simulink model "Appl_HeatAdj_CtrlModel"  (R2018b)
settings: configuration reference "CodeConfig_10_ms" (kept outside this file)
undefined symbols (not defined in the file): CAL_LEVEL3_TIMEOUT, CAL_SW_20min_TIMEOUT, D_1stLevel_36, D_2ndLevel_39, D_3rdLevel_45, D_3rdLevel_48, D_DRVHEAT_PID_D, D_DRVHEAT_PID_I, D_DRVHEAT_PID_P, D_HEAT_HEAT_DEF, D_SwsLevel_Temp, FALSE, TRUE
libraries: DareLib x111, simulink x1
(part 2 of 6)

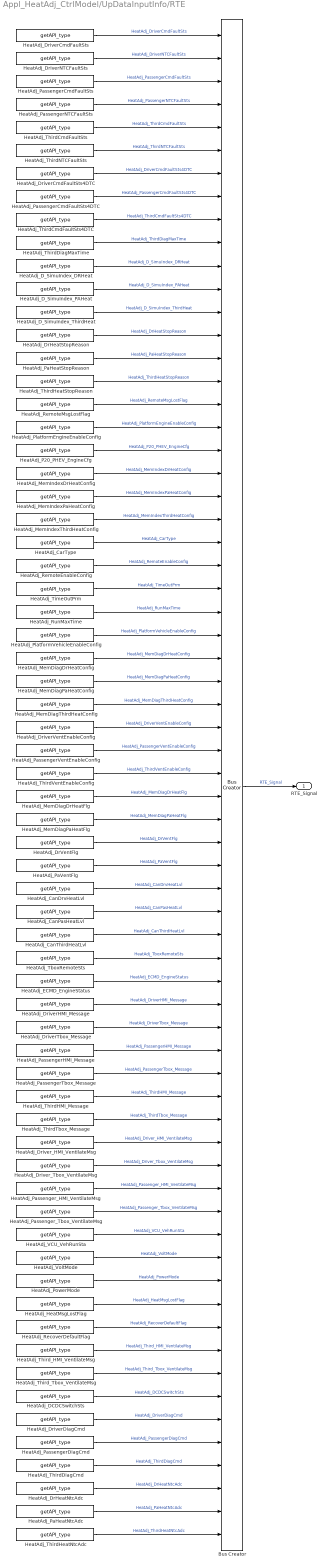
== system Appl_HeatAdj_CtrlModel/UpDataInputInfo/RTE ==
  Bus Creator : BusCreator  Inputs=66
  HeatAdj_CanDrvHeatLvl : DareLib/Dare/getAPI_type  g_funcname=Ecual_CanGetDrvHeatLvl  g_param=""  g_type=uint8  g_size=-1
      settings: AttributesFormatString=%<g_funcname>  SourceProductName=Dare Library
  HeatAdj_CanPasHeatLvl : DareLib/Dare/getAPI_type  g_funcname=Ecual_CanGetPasHeatLvl  g_param=""  g_type=uint8  g_size=-1
      settings: AttributesFormatString=%<g_funcname>  SourceProductName=Dare Library
  HeatAdj_CanThirdHeatLvl : DareLib/Dare/getAPI_type  g_funcname=Ecual_CanGetThirdHeatLvl  g_param=""  g_type=uint8  g_size=-1
      settings: AttributesFormatString=%<g_funcname>  SourceProductName=Dare Library
  HeatAdj_CarType : DareLib/Dare/getAPI_type  g_funcname=Srvl_GetMemIndexDataU8  g_param=EN_MemIndex_Heat_CarType  g_type=uint8  g_enum=enProjectType  g_size=-1
      settings: AttributesFormatString=%<g_funcname>  SourceProductName=Dare Library
  HeatAdj_DCDCSwitchSts : DareLib/Dare/getAPI_type  g_funcname=Vfb_Reserved_0  g_param=""  g_type=uint8  g_size=-1
      settings: AttributesFormatString=%<g_funcname>  SourceProductName=Dare Library
  HeatAdj_D_SimuIndex_DRHeat : DareLib/Dare/getAPI_type  g_funcname=Rte_GetVfb_DrHeat  g_param=""  g_type=uint8  g_enum=enHeatLvlSts  g_size=-1
      settings: AttributesFormatString=%<g_funcname>  SourceProductName=Dare Library
  HeatAdj_D_SimuIndex_PAHeat : DareLib/Dare/getAPI_type  g_funcname=Rte_GetVfb_PaHeat  g_param=""  g_type=uint8  g_enum=enHeatLvlSts  g_size=-1
      settings: AttributesFormatString=%<g_funcname>  SourceProductName=Dare Library
  HeatAdj_D_SimuIndex_ThirdHeat : DareLib/Dare/getAPI_type  g_funcname=Rte_GetVfb_ThirdHeat  g_param=""  g_type=uint8  g_enum=enHeatLvlSts  g_size=-1
      settings: AttributesFormatString=%<g_funcname>  SourceProductName=Dare Library
  HeatAdj_DrHeatNtcAdc : DareLib/Dare/getAPI_type  g_funcname=Ecual_AdcGetDrNTCTempValue  g_param=""  g_type=uint16  g_size=-1
      settings: AttributesFormatString=%<g_funcname>  SourceProductName=Dare Library
  HeatAdj_DrHeatStopReason : DareLib/Dare/getAPI_type  g_funcname=Rte_GetVfb_DrHeatStopReason  g_param=""  g_type=uint8  g_enum=enHeatStopReason  g_size=-1
      settings: AttributesFormatString=%<g_funcname>  SourceProductName=Dare Library
  HeatAdj_DrVentFlg : DareLib/Dare/getAPI_type  g_funcname=Srvl_GetMemIndexDataU8  g_param=EN_MemIndex_DrVentFlg  g_type=uint8  g_size=-1
      settings: AttributesFormatString=%<g_funcname>  SourceProductName=Dare Library
  HeatAdj_DriverCmdFaultSts : DareLib/Dare/getAPI_type  g_funcname=Rte_GetVfb_DrHeatCmdFaultSts  g_param=""  g_type=uint8  g_enum=enHeatCmdFault  g_size=-1
      settings: AttributesFormatString=%<g_funcname>  SourceProductName=Dare Library
  HeatAdj_DriverCmdFaultSts4DTC : DareLib/Dare/getAPI_type  g_funcname=Rte_GetVfb_DrHeatCmdFaultSts4DTC  g_param=""  g_type=uint8  g_enum=enHeatCmdFault  g_size=-1
      settings: AttributesFormatString=%<g_funcname>  SourceProductName=Dare Library
  HeatAdj_DriverDiagCmd : DareLib/Dare/getAPI_type  g_funcname=Desc_DiagOutCtrlPram  g_param=EN_DRHEAT  g_type=uint8  g_enum=enHeatIoCmdLvl  g_size=-1
      settings: AttributesFormatString=%<g_funcname>  SourceProductName=Dare Library
  HeatAdj_DriverHMI_Message : DareLib/Dare/getAPI_type  g_funcname=CanRx_0x351_IVI_FLSeatHeatSet  g_param=""  g_type=uint8  g_size=-1
      settings: AttributesFormatString=%<g_funcname>  SourceProductName=Dare Library
  HeatAdj_DriverNTCFaultSts : DareLib/Dare/getAPI_type  g_funcname=Rte_GetVfb_DrHeatNTCFaultSts  g_param=""  g_type=uint8  g_enum=enHeatNtcFault  g_size=-1
      settings: AttributesFormatString=%<g_funcname>  SourceProductName=Dare Library
  HeatAdj_DriverTbox_Message : DareLib/Dare/getAPI_type  g_funcname=CanRx_0x281_BDC_TBOX_Req_DrSeatHeating  g_param=""  g_type=uint8  g_size=-1
      settings: AttributesFormatString=%<g_funcname>  SourceProductName=Dare Library
  HeatAdj_DriverVentEnableConfig : DareLib/Dare/getAPI_type  g_funcname=Srvl_GetMemIndexDataU8  g_param=EN_MemIndex_DrvVentConfig  g_type=uint8  g_size=-1
      settings: AttributesFormatString=%<g_funcname>  SourceProductName=Dare Library
  HeatAdj_Driver_HMI_VentilateMsg : DareLib/Dare/getAPI_type  g_funcname=CanRx_0x351_IVI_FLSeatVentnSet  g_param=""  g_type=uint8  g_size=-1
      settings: AttributesFormatString=%<g_funcname>  SourceProductName=Dare Library
  HeatAdj_Driver_Tbox_VentilateMsg : DareLib/Dare/getAPI_type  g_funcname=CanRx_0x281_BDC_TBOX_Req_DrSeatVentilating  g_param=""  g_type=uint8  g_size=-1
      settings: AttributesFormatString=%<g_funcname>  SourceProductName=Dare Library
  HeatAdj_ECMD_EngineStatus : DareLib/Dare/getAPI_type  g_funcname=CanRx_0x2A7_ECMD_EngineStatus  g_param=""  g_type=uint8  g_enum=enEngineType  g_size=-1
      settings: AttributesFormatString=%<g_funcname>  SourceProductName=Dare Library
  HeatAdj_HeatMsgLostFlag : DareLib/Dare/getAPI_type  g_funcname=Ecual_CanGetHeatMsgLostFlag  g_param=""  g_type=uint8  g_size=-1
      settings: AttributesFormatString=%<g_funcname>  SourceProductName=Dare Library
  HeatAdj_MemDiagDrHeatConfig : DareLib/Dare/getAPI_type  g_funcname=Srvl_GetMemIndexDataU8  g_param=EN_MemIndex_DrVentAndHeatConfig  g_type=uint8  g_size=-1
      settings: AttributesFormatString=%<g_funcname>  SourceProductName=Dare Library
  HeatAdj_MemDiagDrHeatFlg : DareLib/Dare/getAPI_type  g_funcname=Srvl_GetMemIndexDataU8  g_param=EN_MemIndex_DrHeatFlg  g_type=uint8  g_size=-1
      settings: AttributesFormatString=%<g_funcname>  SourceProductName=Dare Library
  HeatAdj_MemDiagPaHeatConfig : DareLib/Dare/getAPI_type  g_funcname=Srvl_GetMemIndexDataU8  g_param=EN_MemIndex_PaVentAndHeatConfig  g_type=uint8  g_size=-1
      settings: AttributesFormatString=%<g_funcname>  SourceProductName=Dare Library
  HeatAdj_MemDiagPaHeatFlg : DareLib/Dare/getAPI_type  g_funcname=Srvl_GetMemIndexDataU8  g_param=EN_MemIndex_PaHeatFlg  g_type=uint8  g_size=-1
      settings: AttributesFormatString=%<g_funcname>  SourceProductName=Dare Library
  HeatAdj_MemDiagThirdHeatConfig : DareLib/Dare/getAPI_type  g_funcname=Srvl_getSystemConfigPram  g_param=EN_SteerHeat_SysCfg  g_type=uint8  g_size=-1
      settings: AttributesFormatString=%<g_funcname>  SourceProductName=Dare Library
  HeatAdj_MemIndexDrHeatConfig : DareLib/Dare/getAPI_type  g_funcname=Srvl_GetMemIndexDataU8  g_param=EN_MemIndex_DrHeatConfig  g_type=uint8  g_size=-1
      settings: AttributesFormatString=%<g_funcname>  SourceProductName=Dare Library
  HeatAdj_MemIndexPaHeatConfig : DareLib/Dare/getAPI_type  g_funcname=Srvl_GetMemIndexDataU8  g_param=EN_MemIndex_PaHeatFlg  g_type=uint8  g_size=-1
      settings: AttributesFormatString=%<g_funcname>  SourceProductName=Dare Library
  HeatAdj_MemIndexThirdHeatConfig : DareLib/Dare/getAPI_type  g_funcname=Srvl_GetMemIndexDataU8  g_param=EN_MemIndex_ThirdHeatConfig  g_type=uint8  g_size=-1
      settings: AttributesFormatString=%<g_funcname>  SourceProductName=Dare Library
  HeatAdj_P20_PHEV_EngineCfg : DareLib/Dare/getAPI_type  g_funcname=Srvl_GetMemIndexDataU8  g_param=EN_MemIndex_Heat_P20_PHEV_EngineCfg  g_type=uint8  g_size=-1
      settings: AttributesFormatString=%<g_funcname>  SourceProductName=Dare Library
  HeatAdj_PaHeatNtcAdc : DareLib/Dare/getAPI_type  g_funcname=Ecual_AdcGetPaNTCTempValue  g_param=""  g_type=uint16  g_size=-1
      settings: AttributesFormatString=%<g_funcname>  SourceProductName=Dare Library
  HeatAdj_PaHeatStopReason : DareLib/Dare/getAPI_type  g_funcname=Rte_GetVfb_PaHeatStopReason  g_param=""  g_type=uint8  g_enum=enHeatStopReason  g_size=-1
      settings: AttributesFormatString=%<g_funcname>  SourceProductName=Dare Library
  HeatAdj_PaVentFlg : DareLib/Dare/getAPI_type  g_funcname=Srvl_GetMemIndexDataU8  g_param=EN_MemIndex_PaVentFlg  g_type=uint8  g_size=-1
      settings: AttributesFormatString=%<g_funcname>  SourceProductName=Dare Library
  HeatAdj_PassengerCmdFaultSts : DareLib/Dare/getAPI_type  g_funcname=Rte_GetVfb_PaHeatCmdFaultSts  g_param=""  g_type=uint8  g_enum=enHeatCmdFault  g_size=-1
      settings: AttributesFormatString=%<g_funcname>  SourceProductName=Dare Library
  HeatAdj_PassengerCmdFaultSts4DTC : DareLib/Dare/getAPI_type  g_funcname=Rte_GetVfb_PaHeatCmdFaultSts4DTC  g_param=""  g_type=uint8  g_enum=enHeatCmdFault  g_size=-1
      settings: AttributesFormatString=%<g_funcname>  SourceProductName=Dare Library
  HeatAdj_PassengerDiagCmd : DareLib/Dare/getAPI_type  g_funcname=Desc_DiagOutCtrlPram  g_param=EN_PAHEAT  g_type=uint8  g_enum=enHeatIoCmdLvl  g_size=-1
      settings: AttributesFormatString=%<g_funcname>  SourceProductName=Dare Library
  HeatAdj_PassengerHMI_Message : DareLib/Dare/getAPI_type  g_funcname=CanRx_0x351_IVI_FRSeatHeatSet  g_param=""  g_type=uint8  g_size=-1
      settings: AttributesFormatString=%<g_funcname>  SourceProductName=Dare Library
  "HeatAdj_PassengerNTCFaultSts " : DareLib/Dare/getAPI_type  g_funcname=Rte_GetVfb_PaHeatNTCFaultSts  g_param=""  g_type=uint8  g_enum=enHeatNtcFault  g_size=-1
      settings: AttributesFormatString=%<g_funcname>  SourceProductName=Dare Library
  HeatAdj_PassengerTbox_Message : DareLib/Dare/getAPI_type  g_funcname=CanRx_0x281_BDC_TBOX_Req_PaSeatHeating  g_param=""  g_type=uint8  g_size=-1
      settings: AttributesFormatString=%<g_funcname>  SourceProductName=Dare Library
  HeatAdj_PassengerVentEnableConfig : DareLib/Dare/getAPI_type  g_funcname=Srvl_GetMemIndexDataU8  g_param=EN_MemIndex_SecondVentConfig  g_type=uint8  g_size=-1
      settings: AttributesFormatString=%<g_funcname>  SourceProductName=Dare Library
  HeatAdj_Passenger_HMI_VentilateMsg : DareLib/Dare/getAPI_type  g_funcname=CanRx_0x351_IVI_FRSeatVentnSet  g_param=""  g_type=uint8  g_size=-1
      settings: AttributesFormatString=%<g_funcname>  SourceProductName=Dare Library
  HeatAdj_Passenger_Tbox_VentilateMsg : DareLib/Dare/getAPI_type  g_funcname=CanRx_0x281_BDC_TBOX_Req_PaSeatVentilating  g_param=""  g_type=uint8  g_size=-1
      settings: AttributesFormatString=%<g_funcname>  SourceProductName=Dare Library
  HeatAdj_PlatformEngineEnableConfig : DareLib/Dare/getAPI_type  g_funcname=Srvl_GetMemIndexDataU8  g_param=EN_MemIndex_Heat_PlatformEngineEnableConfig  g_type=uint8  g_size=-1
      settings: AttributesFormatString=%<g_funcname>  SourceProductName=Dare Library
  HeatAdj_PlatformVehicleEnableConfig : DareLib/Dare/getAPI_type  g_funcname=Srvl_GetMemIndexDataU8  g_param=EN_MemIndex_Heat_PlatFormVehicleEnableConfig  g_type=uint8  g_size=-1
      settings: AttributesFormatString=%<g_funcname>  SourceProductName=Dare Library
  HeatAdj_PowerMode : DareLib/Dare/getAPI_type  g_funcname=Rte_GetVfb_PowerMode  g_param=""  g_type=uint8  g_enum=enPowerModeSts  g_size=-1
      settings: AttributesFormatString=%<g_funcname>  SourceProductName=Dare Library
  HeatAdj_RecoverDefaultFlag : DareLib/Dare/getAPI_type  g_funcname=GetRecoverDefaultFlag  g_param=""  g_type=uint8  g_size=-1
      settings: AttributesFormatString=%<g_funcname>  SourceProductName=Dare Library
  HeatAdj_RemoteEnableConfig : DareLib/Dare/getAPI_type  g_funcname=Srvl_GetMemIndexDataU8  g_param=EN_MemIndex_Heat_RemoteEnableConfig  g_type=uint8  g_size=-1
      settings: AttributesFormatString=%<g_funcname>  SourceProductName=Dare Library
  HeatAdj_RemoteMsgLostFlag : DareLib/Dare/getAPI_type  g_funcname=Ecual_GetCanMsgLostFlag  g_param=eRXINDEX_0x283  g_type=uint8  g_size=-1
      settings: AttributesFormatString=%<g_funcname>  SourceProductName=Dare Library
  HeatAdj_RunMaxTime : DareLib/Dare/getAPI_type  g_funcname=Srvl_GetMemIndexDataU8  g_param=EN_MemIndex_Heat_RunMaxTime  g_type=uint8  g_size=-1
      settings: AttributesFormatString=%<g_funcname>  SourceProductName=Dare Library
  HeatAdj_TboxRemoteSts : DareLib/Dare/getAPI_type  g_funcname=CanRx_0x283_BDC_TboxRemoteControlSt  g_param=""  g_type=uint8  g_size=-1
      settings: AttributesFormatString=%<g_funcname>  SourceProductName=Dare Library
  HeatAdj_ThirdCmdFaultSts : DareLib/Dare/getAPI_type  g_funcname=Rte_GetVfb_ThirdHeatCmdFaultSts  g_param=""  g_type=uint8  g_enum=enHeatCmdFault  g_size=-1
      settings: AttributesFormatString=%<g_funcname>  SourceProductName=Dare Library
  HeatAdj_ThirdCmdFaultSts4DTC : DareLib/Dare/getAPI_type  g_funcname=Rte_GetVfb_ThirdHeatCmdFaultSts4DTC  g_param=""  g_type=uint8  g_enum=enHeatCmdFault  g_size=-1
      settings: AttributesFormatString=%<g_funcname>  SourceProductName=Dare Library
  HeatAdj_ThirdDiagCmd : DareLib/Dare/getAPI_type  g_funcname=Desc_DiagOutCtrlPram  g_param=EN_WHEEL  g_type=uint8  g_enum=enHeatIoCmdLvl  g_size=-1
      settings: AttributesFormatString=%<g_funcname>  SourceProductName=Dare Library
  HeatAdj_ThirdDiagMaxTime : DareLib/Dare/getAPI_type  g_funcname=Rte_GetVfb_SwHeatMaxTime  g_param=""  g_type=uint8  g_size=-1
      settings: AttributesFormatString=%<g_funcname>  SourceProductName=Dare Library
  HeatAdj_ThirdHMI_Message : DareLib/Dare/getAPI_type  g_funcname=CanRx_0x351_IVI_SwsHeatSw  g_param=""  g_type=uint8  g_size=-1
      settings: AttributesFormatString=%<g_funcname>  SourceProductName=Dare Library
  HeatAdj_ThirdHeatNtcAdc : DareLib/Dare/getAPI_type  g_funcname=Ecual_AdcGetCenterNTCTempValue  g_param=""  g_type=uint16  g_size=-1
      settings: AttributesFormatString=%<g_funcname>  SourceProductName=Dare Library
  "HeatAdj_ThirdHeatStopReason " : DareLib/Dare/getAPI_type  g_funcname=Rte_GetVfb_ThirdHeatStopReason  g_param=""  g_type=uint8  g_enum=enHeatStopReason  g_size=-1
      settings: AttributesFormatString=%<g_funcname>  SourceProductName=Dare Library
  HeatAdj_ThirdNTCFaultSts : DareLib/Dare/getAPI_type  g_funcname=Rte_GetVfb_ThirdHeatNTCFaultSts  g_param=""  g_type=uint8  g_enum=enHeatNtcFault  g_size=-1
      settings: AttributesFormatString=%<g_funcname>  SourceProductName=Dare Library
  HeatAdj_ThirdTbox_Message : DareLib/Dare/getAPI_type  g_funcname=CanRx_0x281_BDC_TBOX_Req_Steeringwheel_heating  g_param=""  g_type=uint8  g_size=-1
      settings: AttributesFormatString=%<g_funcname>  SourceProductName=Dare Library
  HeatAdj_ThirdVentEnableConfig : DareLib/Dare/getAPI_type  g_funcname=Srvl_GetMemIndexDataU8  g_param=EN_MemIndex_ThirdVentConfig  g_type=uint8  g_size=-1
      settings: AttributesFormatString=%<g_funcname>  SourceProductName=Dare Library
  HeatAdj_Third_HMI_VentilateMsg : DareLib/Dare/getAPI_type  g_funcname=Vfb_Reserved_0  g_param=""  g_type=uint8  g_size=-1
      settings: AttributesFormatString=%<g_funcname>  SourceProductName=Dare Library
  HeatAdj_Third_Tbox_VentilateMsg : DareLib/Dare/getAPI_type  g_funcname=Vfb_Reserved_0  g_param=""  g_type=uint8  g_size=-1
      settings: AttributesFormatString=%<g_funcname>  SourceProductName=Dare Library
  HeatAdj_TimeOutPrm : DareLib/Dare/getAPI_type  g_funcname=Srvl_GetMemIndexDataU8  g_param=EN_MemIndex_Heat_TimeOutPrm  g_type=uint8  g_size=-1
      settings: AttributesFormatString=%<g_funcname>  SourceProductName=Dare Library
  HeatAdj_VCU_VehRunSta : DareLib/Dare/getAPI_type  g_funcname=CanRx_0x2AE_VCU_VehRunSta  g_param=""  g_type=uint8  g_enum=enVehicleRunType  g_size=-1
      settings: AttributesFormatString=%<g_funcname>  SourceProductName=Dare Library
  HeatAdj_VoltMode : DareLib/Dare/getAPI_type  g_funcname=Rte_GetVfb_VoltMode  g_param=""  g_type=uint8  g_enum=enFinalPowerMode  g_size=-1
      settings: AttributesFormatString=%<g_funcname>  SourceProductName=Dare Library
  RTE_Signal : Outport
  wires:
  Bus Creator/1 -> RTE_Signal/1  "RTE_Signal"
  HeatAdj_DriverCmdFaultSts/1 -> Bus Creator/1  "HeatAdj_DriverCmdFaultSts"
  HeatAdj_DriverNTCFaultSts/1 -> Bus Creator/2  "HeatAdj_DriverNTCFaultSts"
  HeatAdj_PassengerCmdFaultSts/1 -> Bus Creator/3  "HeatAdj_PassengerCmdFaultSts"
  "HeatAdj_PassengerNTCFaultSts "/1 -> Bus Creator/4  "HeatAdj_PassengerNTCFaultSts"
  HeatAdj_ThirdCmdFaultSts/1 -> Bus Creator/5  "HeatAdj_ThirdCmdFaultSts"
  HeatAdj_ThirdNTCFaultSts/1 -> Bus Creator/6  "HeatAdj_ThirdNTCFaultSts"
  HeatAdj_DriverCmdFaultSts4DTC/1 -> Bus Creator/7  "HeatAdj_DriverCmdFaultSts4DTC"
  HeatAdj_PassengerCmdFaultSts4DTC/1 -> Bus Creator/8  "HeatAdj_PassengerCmdFaultSts4DTC"
  HeatAdj_ThirdCmdFaultSts4DTC/1 -> Bus Creator/9  "HeatAdj_ThirdCmdFaultSts4DTC"
  HeatAdj_ThirdDiagMaxTime/1 -> Bus Creator/10  "HeatAdj_ThirdDiagMaxTime"
  HeatAdj_D_SimuIndex_DRHeat/1 -> Bus Creator/11  "HeatAdj_D_SimuIndex_DRHeat"
  HeatAdj_D_SimuIndex_PAHeat/1 -> Bus Creator/12  "HeatAdj_D_SimuIndex_PAHeat"
  HeatAdj_D_SimuIndex_ThirdHeat/1 -> Bus Creator/13  "HeatAdj_D_SimuIndex_ThirdHeat"
  HeatAdj_DrHeatStopReason/1 -> Bus Creator/14  "HeatAdj_DrHeatStopReason"
  HeatAdj_PaHeatStopReason/1 -> Bus Creator/15  "HeatAdj_PaHeatStopReason"
  "HeatAdj_ThirdHeatStopReason "/1 -> Bus Creator/16  "HeatAdj_ThirdHeatStopReason"
  HeatAdj_RemoteMsgLostFlag/1 -> Bus Creator/17  "HeatAdj_RemoteMsgLostFlag"
  HeatAdj_PlatformEngineEnableConfig/1 -> Bus Creator/18  "HeatAdj_PlatformEngineEnableConfig"
  HeatAdj_P20_PHEV_EngineCfg/1 -> Bus Creator/19  "HeatAdj_P20_PHEV_EngineCfg"
  HeatAdj_MemIndexDrHeatConfig/1 -> Bus Creator/20  "HeatAdj_MemIndexDrHeatConfig"
  HeatAdj_MemIndexPaHeatConfig/1 -> Bus Creator/21  "HeatAdj_MemIndexPaHeatConfig"
  HeatAdj_MemIndexThirdHeatConfig/1 -> Bus Creator/22  "HeatAdj_MemIndexThirdHeatConfig"
  HeatAdj_CarType/1 -> Bus Creator/23  "HeatAdj_CarType"
  HeatAdj_RemoteEnableConfig/1 -> Bus Creator/24  "HeatAdj_RemoteEnableConfig"
  HeatAdj_TimeOutPrm/1 -> Bus Creator/25  "HeatAdj_TimeOutPrm"
  HeatAdj_RunMaxTime/1 -> Bus Creator/26  "HeatAdj_RunMaxTime"
  HeatAdj_PlatformVehicleEnableConfig/1 -> Bus Creator/27  "HeatAdj_PlatformVehicleEnableConfig"
  HeatAdj_MemDiagDrHeatConfig/1 -> Bus Creator/28  "HeatAdj_MemDiagDrHeatConfig"
  HeatAdj_MemDiagPaHeatConfig/1 -> Bus Creator/29  "HeatAdj_MemDiagPaHeatConfig"
  HeatAdj_MemDiagThirdHeatConfig/1 -> Bus Creator/30  "HeatAdj_MemDiagThirdHeatConfig"
  HeatAdj_DriverVentEnableConfig/1 -> Bus Creator/31  "HeatAdj_DriverVentEnableConfig"
  HeatAdj_PassengerVentEnableConfig/1 -> Bus Creator/32  "HeatAdj_PassengerVentEnableConfig"
  HeatAdj_ThirdVentEnableConfig/1 -> Bus Creator/33  "HeatAdj_ThirdVentEnableConfig"
  HeatAdj_MemDiagDrHeatFlg/1 -> Bus Creator/34  "HeatAdj_MemDiagDrHeatFlg"
  HeatAdj_MemDiagPaHeatFlg/1 -> Bus Creator/35  "HeatAdj_MemDiagPaHeatFlg"
  HeatAdj_DrVentFlg/1 -> Bus Creator/36  "HeatAdj_DrVentFlg"
  HeatAdj_PaVentFlg/1 -> Bus Creator/37  "HeatAdj_PaVentFlg"
  HeatAdj_CanDrvHeatLvl/1 -> Bus Creator/38  "HeatAdj_CanDrvHeatLvl"
  HeatAdj_CanPasHeatLvl/1 -> Bus Creator/39  "HeatAdj_CanPasHeatLvl"
  HeatAdj_CanThirdHeatLvl/1 -> Bus Creator/40  "HeatAdj_CanThirdHeatLvl"
  HeatAdj_TboxRemoteSts/1 -> Bus Creator/41  "HeatAdj_TboxRemoteSts"
  HeatAdj_ECMD_EngineStatus/1 -> Bus Creator/42  "HeatAdj_ECMD_EngineStatus"
  HeatAdj_DriverHMI_Message/1 -> Bus Creator/43  "HeatAdj_DriverHMI_Message"
  HeatAdj_DriverTbox_Message/1 -> Bus Creator/44  "HeatAdj_DriverTbox_Message"
  HeatAdj_PassengerHMI_Message/1 -> Bus Creator/45  "HeatAdj_PassengerHMI_Message"
  HeatAdj_PassengerTbox_Message/1 -> Bus Creator/46  "HeatAdj_PassengerTbox_Message"
  HeatAdj_ThirdHMI_Message/1 -> Bus Creator/47  "HeatAdj_ThirdHMI_Message"
  HeatAdj_ThirdTbox_Message/1 -> Bus Creator/48  "HeatAdj_ThirdTbox_Message"
  HeatAdj_Driver_HMI_VentilateMsg/1 -> Bus Creator/49  "HeatAdj_Driver_HMI_VentilateMsg"
  HeatAdj_Driver_Tbox_VentilateMsg/1 -> Bus Creator/50  "HeatAdj_Driver_Tbox_VentilateMsg"
  HeatAdj_Passenger_HMI_VentilateMsg/1 -> Bus Creator/51  "HeatAdj_Passenger_HMI_VentilateMsg"
  HeatAdj_Passenger_Tbox_VentilateMsg/1 -> Bus Creator/52  "HeatAdj_Passenger_Tbox_VentilateMsg"
  HeatAdj_VCU_VehRunSta/1 -> Bus Creator/53  "HeatAdj_VCU_VehRunSta"
  HeatAdj_VoltMode/1 -> Bus Creator/54  "HeatAdj_VoltMode"
  HeatAdj_PowerMode/1 -> Bus Creator/55  "HeatAdj_PowerMode"
  HeatAdj_HeatMsgLostFlag/1 -> Bus Creator/56  "HeatAdj_HeatMsgLostFlag"
  HeatAdj_RecoverDefaultFlag/1 -> Bus Creator/57  "HeatAdj_RecoverDefaultFlag"
  HeatAdj_Third_HMI_VentilateMsg/1 -> Bus Creator/58  "HeatAdj_Third_HMI_VentilateMsg"
  HeatAdj_Third_Tbox_VentilateMsg/1 -> Bus Creator/59  "HeatAdj_Third_Tbox_VentilateMsg"
  HeatAdj_DCDCSwitchSts/1 -> Bus Creator/60  "HeatAdj_DCDCSwitchSts"
  HeatAdj_DriverDiagCmd/1 -> Bus Creator/61  "HeatAdj_DriverDiagCmd"
  HeatAdj_PassengerDiagCmd/1 -> Bus Creator/62  "HeatAdj_PassengerDiagCmd"
  HeatAdj_ThirdDiagCmd/1 -> Bus Creator/63  "HeatAdj_ThirdDiagCmd"
  HeatAdj_DrHeatNtcAdc/1 -> Bus Creator/64  "HeatAdj_DrHeatNtcAdc"
  HeatAdj_PaHeatNtcAdc/1 -> Bus Creator/65  "HeatAdj_PaHeatNtcAdc"
  HeatAdj_ThirdHeatNtcAdc/1 -> Bus Creator/66  "HeatAdj_ThirdHeatNtcAdc"

== system Appl_HeatAdj_CtrlModel/LogicCtrl/LocalAdjustCtrl/HeatLevelDeal/CANAquireFunction ==
  HeatLevel : Inport
  IVISwsHeat : Inport  Port=2
  PowerMode : Inport  Port=3
  f : TriggerPort  TriggerType=function-call  VariantControl=(inherit)
      settings: CopyFcn=Stateflow.SLINSF.SimulinkMan.removeBlockPreDeleteFcn  PreDeleteFcn=Stateflow.SLINSF.SimulinkMan.unsafePredeleteFcn
  CANAquireFunction : Stateflow chart  TreatAsAtomicUnit=on
  "IVISwCan " : Outport
  wires:
  HeatLevel/1 -> CANAquireFunction/1(HeatLevel)
  IVISwsHeat/1 -> CANAquireFunction/2(IVISwsHeat)
  PowerMode/1 -> CANAquireFunction/3(PowerMode)
  CANAquireFunction/1(IVISwCan) -> "IVISwCan "/1

== system Appl_HeatAdj_CtrlModel/LogicCtrl/LocalAdjustCtrl/HeatLevelDeal/LevelAquireFunction ==
  EnableCfg : Inport
  CarTypeCfg : Inport  Port=2
  CAN_Message : Inport  Port=3
  DisableSts : Inport  Port=4
  ComPCFlag : Inport  Port=5  OutDataTypeStr=uint8
  CanLvl : Inport  Port=6  OutDataTypeStr=uint8
  Type : Inport  Port=7  OutDataTypeStr=uint8
  f : TriggerPort  TriggerType=function-call  VariantControl=(inherit)
      settings: CopyFcn=Stateflow.SLINSF.SimulinkMan.removeBlockPreDeleteFcn  PreDeleteFcn=Stateflow.SLINSF.SimulinkMan.unsafePredeleteFcn
  LevelAquireFunction : Stateflow chart  TreatAsAtomicUnit=on
  "Level " : Outport
  wires:
  EnableCfg/1 -> LevelAquireFunction/1(EnableCfg)
  DisableSts/1 -> LevelAquireFunction/4(DisableSts)
  CarTypeCfg/1 -> LevelAquireFunction/2(CarTypeCfg)
  CAN_Message/1 -> LevelAquireFunction/3(CAN_Message)
  LevelAquireFunction/1(Level) -> "Level "/1
  ComPCFlag/1 -> LevelAquireFunction/5(ComPCFlag)
  CanLvl/1 -> LevelAquireFunction/6(CanLvl)
  Type/1 -> LevelAquireFunction/7(Type)
  ? -> LevelAquireFunction/8(CurLvl)

== system Appl_HeatAdj_CtrlModel/LogicCtrl/LocalAdjustCtrl/HeatLevelDeal/LevelAquireFunction1 ==
  EnableCfg : Inport
  CarTypeCfg : Inport  Port=2
  CAN_Message : Inport  Port=3
  DisableSts : Inport  Port=4
  ComPCFlag : Inport  Port=5  OutDataTypeStr=uint8
  CanLvl : Inport  Port=6  OutDataTypeStr=uint8
  Type : Inport  Port=7  OutDataTypeStr=uint8
  f : TriggerPort  TriggerType=function-call  VariantControl=(inherit)
      settings: CopyFcn=Stateflow.SLINSF.SimulinkMan.removeBlockPreDeleteFcn  PreDeleteFcn=Stateflow.SLINSF.SimulinkMan.unsafePredeleteFcn
  LevelAquireFunction : Stateflow chart  TreatAsAtomicUnit=on
  "Level " : Outport
  wires:
  EnableCfg/1 -> LevelAquireFunction/1(EnableCfg)
  DisableSts/1 -> LevelAquireFunction/4(DisableSts)
  CarTypeCfg/1 -> LevelAquireFunction/2(CarTypeCfg)
  CAN_Message/1 -> LevelAquireFunction/3(CAN_Message)
  LevelAquireFunction/1(Level) -> "Level "/1
  ComPCFlag/1 -> LevelAquireFunction/5(ComPCFlag)
  CanLvl/1 -> LevelAquireFunction/6(CanLvl)
  Type/1 -> LevelAquireFunction/7(Type)
  ? -> LevelAquireFunction/8(CurLvl)

== system Appl_HeatAdj_CtrlModel/LogicCtrl/LocalAdjustCtrl/HeatLevelDeal/LevelAquireFunction2 ==
  EnableCfg : Inport
  CarTypeCfg : Inport  Port=2
  CAN_Message : Inport  Port=3
  DisableSts : Inport  Port=4
  ComPCFlag : Inport  Port=5  OutDataTypeStr=uint8
  CanLvl : Inport  Port=6  OutDataTypeStr=uint8
  Type : Inport  Port=7  OutDataTypeStr=uint8
  f : TriggerPort  TriggerType=function-call  VariantControl=(inherit)
      settings: CopyFcn=Stateflow.SLINSF.SimulinkMan.removeBlockPreDeleteFcn  PreDeleteFcn=Stateflow.SLINSF.SimulinkMan.unsafePredeleteFcn
  LevelAquireFunction : Stateflow chart  TreatAsAtomicUnit=on
  "Level " : Outport
  wires:
  EnableCfg/1 -> LevelAquireFunction/1(EnableCfg)
  DisableSts/1 -> LevelAquireFunction/4(DisableSts)
  CarTypeCfg/1 -> LevelAquireFunction/2(CarTypeCfg)
  CAN_Message/1 -> LevelAquireFunction/3(CAN_Message)
  LevelAquireFunction/1(Level) -> "Level "/1
  ComPCFlag/1 -> LevelAquireFunction/5(ComPCFlag)
  CanLvl/1 -> LevelAquireFunction/6(CanLvl)
  Type/1 -> LevelAquireFunction/7(Type)
  ? -> LevelAquireFunction/8(CurLvl)

== system Appl_HeatAdj_CtrlModel/LogicCtrl/LocalAdjustCtrl/HeatLevelDeal/LevelAquireFunction3 ==
  EnableCfg : Inport
  CarTypeCfg : Inport  Port=2
  CAN_Message : Inport  Port=3
  DisableSts : Inport  Port=4
  ComPCFlag : Inport  Port=5  OutDataTypeStr=uint8
  CanLvl : Inport  Port=6  OutDataTypeStr=uint8
  Type : Inport  Port=7  OutDataTypeStr=uint8
  f : TriggerPort  TriggerType=function-call  VariantControl=(inherit)
      settings: CopyFcn=Stateflow.SLINSF.SimulinkMan.removeBlockPreDeleteFcn  PreDeleteFcn=Stateflow.SLINSF.SimulinkMan.unsafePredeleteFcn
  LevelAquireFunction : Stateflow chart  TreatAsAtomicUnit=on
  "Level " : Outport
  wires:
  EnableCfg/1 -> LevelAquireFunction/1(EnableCfg)
  DisableSts/1 -> LevelAquireFunction/4(DisableSts)
  CarTypeCfg/1 -> LevelAquireFunction/2(CarTypeCfg)
  CAN_Message/1 -> LevelAquireFunction/3(CAN_Message)
  LevelAquireFunction/1(Level) -> "Level "/1
  ComPCFlag/1 -> LevelAquireFunction/5(ComPCFlag)
  CanLvl/1 -> LevelAquireFunction/6(CanLvl)
  Type/1 -> LevelAquireFunction/7(Type)
  ? -> LevelAquireFunction/8(CurLvl)

== system Appl_HeatAdj_CtrlModel/LogicCtrl/LocalAdjustCtrl/HeatLevelDeal/LevelAquireFunction4 ==
  EnableCfg : Inport
  CarTypeCfg : Inport  Port=2
  CAN_Message : Inport  Port=3
  DisableSts : Inport  Port=4
  ComPCFlag : Inport  Port=5  OutDataTypeStr=uint8
  CanLvl : Inport  Port=6  OutDataTypeStr=uint8
  Type : Inport  Port=7  OutDataTypeStr=uint8
  f : TriggerPort  TriggerType=function-call  VariantControl=(inherit)
      settings: CopyFcn=Stateflow.SLINSF.SimulinkMan.removeBlockPreDeleteFcn  PreDeleteFcn=Stateflow.SLINSF.SimulinkMan.unsafePredeleteFcn
  LevelAquireFunction : Stateflow chart  TreatAsAtomicUnit=on
  "Level " : Outport
  wires:
  EnableCfg/1 -> LevelAquireFunction/1(EnableCfg)
  DisableSts/1 -> LevelAquireFunction/4(DisableSts)
  CarTypeCfg/1 -> LevelAquireFunction/2(CarTypeCfg)
  CAN_Message/1 -> LevelAquireFunction/3(CAN_Message)
  LevelAquireFunction/1(Level) -> "Level "/1
  ComPCFlag/1 -> LevelAquireFunction/5(ComPCFlag)
  CanLvl/1 -> LevelAquireFunction/6(CanLvl)
  Type/1 -> LevelAquireFunction/7(Type)
  ? -> LevelAquireFunction/8(CurLvl)

== system Appl_HeatAdj_CtrlModel/LogicCtrl/LocalAdjustCtrl/HeatLevelDeal/LevelAquireFunction5 ==
  EnableCfg : Inport
  CarTypeCfg : Inport  Port=2
  CAN_Message : Inport  Port=3
  DisableSts : Inport  Port=4
  ComPCFlag : Inport  Port=5  OutDataTypeStr=uint8
  CanLvl : Inport  Port=6  OutDataTypeStr=uint8
  Type : Inport  Port=7  OutDataTypeStr=uint8
  f : TriggerPort  TriggerType=function-call  VariantControl=(inherit)
      settings: CopyFcn=Stateflow.SLINSF.SimulinkMan.removeBlockPreDeleteFcn  PreDeleteFcn=Stateflow.SLINSF.SimulinkMan.unsafePredeleteFcn
  LevelAquireFunction : Stateflow chart  TreatAsAtomicUnit=on
  "Level " : Outport
  wires:
  EnableCfg/1 -> LevelAquireFunction/1(EnableCfg)
  DisableSts/1 -> LevelAquireFunction/4(DisableSts)
  CarTypeCfg/1 -> LevelAquireFunction/2(CarTypeCfg)
  CAN_Message/1 -> LevelAquireFunction/3(CAN_Message)
  LevelAquireFunction/1(Level) -> "Level "/1
  ComPCFlag/1 -> LevelAquireFunction/5(ComPCFlag)
  CanLvl/1 -> LevelAquireFunction/6(CanLvl)
  Type/1 -> LevelAquireFunction/7(Type)
  ? -> LevelAquireFunction/8(CurLvl)

== system Appl_HeatAdj_CtrlModel/LogicCtrl/LocalAdjustCtrl/HeatLevelDeal/SwLevelAquireFunction ==
  EnableCfg : Inport
  CAN_Message : Inport  Port=2
  DisableSts : Inport  Port=3
  ComPCFlag : Inport  Port=4  OutDataTypeStr=uint8
  f : TriggerPort  TriggerType=function-call  VariantControl=(inherit)
      settings: CopyFcn=Stateflow.SLINSF.SimulinkMan.removeBlockPreDeleteFcn  PreDeleteFcn=Stateflow.SLINSF.SimulinkMan.unsafePredeleteFcn
  SwLevelAquireFunction : Stateflow chart  TreatAsAtomicUnit=on
  "Level " : Outport
  wires:
  EnableCfg/1 -> SwLevelAquireFunction/1(EnableCfg)
  DisableSts/1 -> SwLevelAquireFunction/3(DisableSts)
  CAN_Message/1 -> SwLevelAquireFunction/2(CAN_Message)
  SwLevelAquireFunction/1(Level) -> "Level "/1
  ComPCFlag/1 -> SwLevelAquireFunction/4(ComPCFlag)

== system Appl_HeatAdj_CtrlModel/LogicCtrl/LocalAdjustCtrl/HeatLevelDeal/SwLevelAquireFunction1 ==
  EnableCfg : Inport
  CAN_Message : Inport  Port=2
  DisableSts : Inport  Port=3
  ComPCFlag : Inport  Port=4  OutDataTypeStr=uint8
  f : TriggerPort  TriggerType=function-call  VariantControl=(inherit)
      settings: CopyFcn=Stateflow.SLINSF.SimulinkMan.removeBlockPreDeleteFcn  PreDeleteFcn=Stateflow.SLINSF.SimulinkMan.unsafePredeleteFcn
  SwLevelAquireFunction : Stateflow chart  TreatAsAtomicUnit=on
  "Level " : Outport
  wires:
  EnableCfg/1 -> SwLevelAquireFunction/1(EnableCfg)
  DisableSts/1 -> SwLevelAquireFunction/3(DisableSts)
  CAN_Message/1 -> SwLevelAquireFunction/2(CAN_Message)
  SwLevelAquireFunction/1(Level) -> "Level "/1
  ComPCFlag/1 -> SwLevelAquireFunction/4(ComPCFlag)

== system Appl_HeatAdj_CtrlModel/LogicCtrl/LocalAdjustCtrl/LimitDeal/DiagnoseFunction ==
  DiagCommand : Inport
  InLevel : Inport  Port=2
  CurrentType : Inport  Port=3
  f : TriggerPort  TriggerType=function-call  VariantControl=(inherit)
      settings: CopyFcn=Stateflow.SLINSF.SimulinkMan.removeBlockPreDeleteFcn  PreDeleteFcn=Stateflow.SLINSF.SimulinkMan.unsafePredeleteFcn
  Diagnose : Stateflow chart  TreatAsAtomicUnit=on
  Level : Outport
  Type : Outport  Port=2
  wires:
  DiagCommand/1 -> Diagnose/1(DiagCommand)
  InLevel/1 -> Diagnose/2(InLevel)
  CurrentType/1 -> Diagnose/3(CurrentType)
  Diagnose/1(Level) -> Level/1
  Diagnose/2(Type) -> Type/1

== system Appl_HeatAdj_CtrlModel/LogicCtrl/LocalAdjustCtrl/LimitDeal/DiagnoseFunction1 ==
  DiagCommand : Inport
  InLevel : Inport  Port=2
  CurrentType : Inport  Port=3
  f : TriggerPort  TriggerType=function-call  VariantControl=(inherit)
      settings: CopyFcn=Stateflow.SLINSF.SimulinkMan.removeBlockPreDeleteFcn  PreDeleteFcn=Stateflow.SLINSF.SimulinkMan.unsafePredeleteFcn
  Diagnose : Stateflow chart  TreatAsAtomicUnit=on
  Level : Outport
  Type : Outport  Port=2
  wires:
  DiagCommand/1 -> Diagnose/1(DiagCommand)
  InLevel/1 -> Diagnose/2(InLevel)
  CurrentType/1 -> Diagnose/3(CurrentType)
  Diagnose/1(Level) -> Level/1
  Diagnose/2(Type) -> Type/1

== system Appl_HeatAdj_CtrlModel/LogicCtrl/LocalAdjustCtrl/LimitDeal/DiagnoseFunction2 ==
  DiagCommand : Inport
  InLevel : Inport  Port=2
  CurrentType : Inport  Port=3
  f : TriggerPort  TriggerType=function-call  VariantControl=(inherit)
      settings: CopyFcn=Stateflow.SLINSF.SimulinkMan.removeBlockPreDeleteFcn  PreDeleteFcn=Stateflow.SLINSF.SimulinkMan.unsafePredeleteFcn
  Diagnose : Stateflow chart  TreatAsAtomicUnit=on
  Level : Outport
  Type : Outport  Port=2
  wires:
  DiagCommand/1 -> Diagnose/1(DiagCommand)
  InLevel/1 -> Diagnose/2(InLevel)
  CurrentType/1 -> Diagnose/3(CurrentType)
  Diagnose/1(Level) -> Level/1
  Diagnose/2(Type) -> Type/1

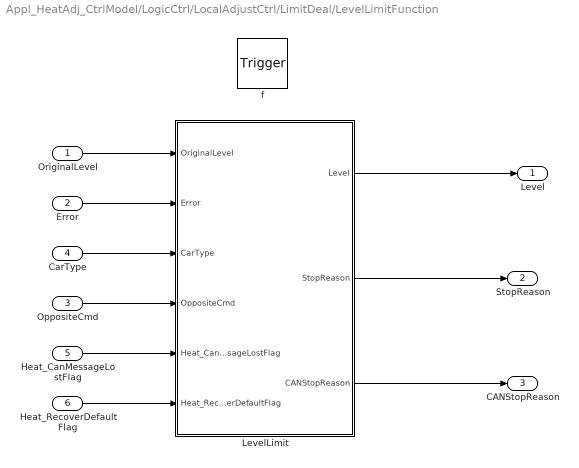
== system Appl_HeatAdj_CtrlModel/LogicCtrl/LocalAdjustCtrl/LimitDeal/LevelLimitFunction ==
  OriginalLevel : Inport
  Error : Inport  Port=2
  OppositeCmd : Inport  Port=3
  CarType : Inport  Port=4
  Heat_CanMessageLostFlag : Inport  Port=5
  Heat_RecoverDefaultFlag : Inport  Port=6
  f : TriggerPort  TriggerType=function-call  VariantControl=(inherit)
      settings: CopyFcn=Stateflow.SLINSF.SimulinkMan.removeBlockPreDeleteFcn  PreDeleteFcn=Stateflow.SLINSF.SimulinkMan.unsafePredeleteFcn
  LevelLimit : Stateflow chart  TreatAsAtomicUnit=on
  Level : Outport
  StopReason : Outport  Port=2
  CANStopReason : Outport  Port=3
  wires:
  OriginalLevel/1 -> LevelLimit/1(OriginalLevel)
  Error/1 -> LevelLimit/2(Error)
  CarType/1 -> LevelLimit/3(CarType)
  OppositeCmd/1 -> LevelLimit/4(OppositeCmd)
  Heat_CanMessageLostFlag/1 -> LevelLimit/5(Heat_CanMessageLostFlag)
  Heat_RecoverDefaultFlag/1 -> LevelLimit/6(Heat_RecoverDefaultFlag)
  LevelLimit/1(Level) -> Level/1
  LevelLimit/2(StopReason) -> StopReason/1
  LevelLimit/3(CANStopReason) -> CANStopReason/1

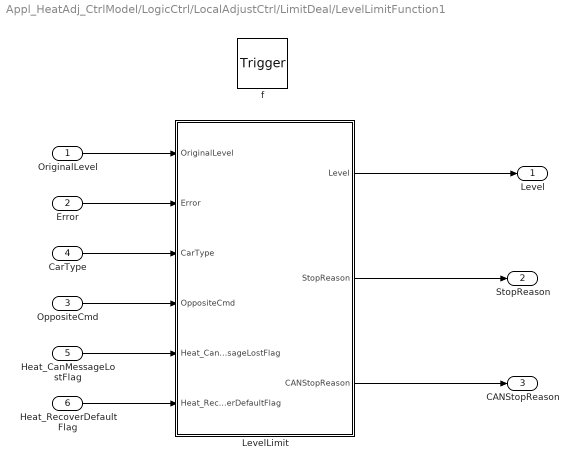
== system Appl_HeatAdj_CtrlModel/LogicCtrl/LocalAdjustCtrl/LimitDeal/LevelLimitFunction1 ==
  OriginalLevel : Inport
  Error : Inport  Port=2
  OppositeCmd : Inport  Port=3
  CarType : Inport  Port=4
  Heat_CanMessageLostFlag : Inport  Port=5
  Heat_RecoverDefaultFlag : Inport  Port=6
  f : TriggerPort  TriggerType=function-call  VariantControl=(inherit)
      settings: CopyFcn=Stateflow.SLINSF.SimulinkMan.removeBlockPreDeleteFcn  PreDeleteFcn=Stateflow.SLINSF.SimulinkMan.unsafePredeleteFcn
  LevelLimit : Stateflow chart  TreatAsAtomicUnit=on
  Level : Outport
  StopReason : Outport  Port=2
  CANStopReason : Outport  Port=3
  wires:
  OriginalLevel/1 -> LevelLimit/1(OriginalLevel)
  Error/1 -> LevelLimit/2(Error)
  CarType/1 -> LevelLimit/3(CarType)
  OppositeCmd/1 -> LevelLimit/4(OppositeCmd)
  Heat_CanMessageLostFlag/1 -> LevelLimit/5(Heat_CanMessageLostFlag)
  Heat_RecoverDefaultFlag/1 -> LevelLimit/6(Heat_RecoverDefaultFlag)
  LevelLimit/1(Level) -> Level/1
  LevelLimit/2(StopReason) -> StopReason/1
  LevelLimit/3(CANStopReason) -> CANStopReason/1

== system Appl_HeatAdj_CtrlModel/LogicCtrl/LocalAdjustCtrl/LimitDeal/LevelLimitFunction2 ==
  OriginalLevel : Inport
  Error : Inport  Port=2
  OppositeCmd : Inport  Port=3
  CarType : Inport  Port=4
  Heat_CanMessageLostFlag : Inport  Port=5
  Heat_RecoverDefaultFlag : Inport  Port=6
  f : TriggerPort  TriggerType=function-call  VariantControl=(inherit)
      settings: CopyFcn=Stateflow.SLINSF.SimulinkMan.removeBlockPreDeleteFcn  PreDeleteFcn=Stateflow.SLINSF.SimulinkMan.unsafePredeleteFcn
  LevelLimit : Stateflow chart  TreatAsAtomicUnit=on
  Level : Outport
  StopReason : Outport  Port=2
  CANStopReason : Outport  Port=3
  wires:
  OriginalLevel/1 -> LevelLimit/1(OriginalLevel)
  Error/1 -> LevelLimit/2(Error)
  CarType/1 -> LevelLimit/3(CarType)
  OppositeCmd/1 -> LevelLimit/4(OppositeCmd)
  Heat_CanMessageLostFlag/1 -> LevelLimit/5(Heat_CanMessageLostFlag)
  Heat_RecoverDefaultFlag/1 -> LevelLimit/6(Heat_RecoverDefaultFlag)
  LevelLimit/1(Level) -> Level/1
  LevelLimit/2(StopReason) -> StopReason/1
  LevelLimit/3(CANStopReason) -> CANStopReason/1

== system Appl_HeatAdj_CtrlModel/LogicCtrl/LocalAdjustCtrl/LimitDeal/MixConflic ==
  MixFlg : Inport  OutDataTypeStr=uint8
  Valid : Inport  Port=2  OutDataTypeStr=uint8
  f : TriggerPort  TriggerType=function-call  VariantControl=(inherit)
      settings: CopyFcn=Stateflow.SLINSF.SimulinkMan.removeBlockPreDeleteFcn  PreDeleteFcn=Stateflow.SLINSF.SimulinkMan.unsafePredeleteFcn
  Constant : Constant  Value=FALSE
  Switch : Switch  Criteria=u2 ~= 0  OutDataTypeStr=uint8
  OutValid : Outport
  wires:
  MixFlg/1 -> Switch/2
  Constant/1 -> Switch/1
  Valid/1 -> Switch/3
  Switch/1 -> OutValid/1

== system Appl_HeatAdj_CtrlModel/LogicCtrl/LocalAdjustCtrl/LimitDeal/StopFunction ==
  ComStop : Inport
  Timeout : Inport  Port=2
  ComCANStop : Inport  Port=3  OutDataTypeStr=Enum: enHeatStopReason
  f : TriggerPort  TriggerType=function-call  VariantControl=(inherit)
      settings: CopyFcn=Stateflow.SLINSF.SimulinkMan.removeBlockPreDeleteFcn  PreDeleteFcn=Stateflow.SLINSF.SimulinkMan.unsafePredeleteFcn
  StopFunction : Stateflow chart  TreatAsAtomicUnit=on
  StopReason : Outport
  CANStopReason : Outport  Port=2
  wires:
  Timeout/1 -> StopFunction/2(Timeout)
  ComStop/1 -> StopFunction/1(ComStop)
  StopFunction/1(StopReason) -> StopReason/1
  ComCANStop/1 -> StopFunction/3(ComCANStop)
  StopFunction/2(CANStopReason) -> CANStopReason/1

== system Appl_HeatAdj_CtrlModel/LogicCtrl/LocalAdjustCtrl/LimitDeal/StopFunction1 ==
  ComStop : Inport
  Timeout : Inport  Port=2
  ComCANStop : Inport  Port=3  OutDataTypeStr=Enum: enHeatStopReason
  f : TriggerPort  TriggerType=function-call  VariantControl=(inherit)
      settings: CopyFcn=Stateflow.SLINSF.SimulinkMan.removeBlockPreDeleteFcn  PreDeleteFcn=Stateflow.SLINSF.SimulinkMan.unsafePredeleteFcn
  StopFunction : Stateflow chart  TreatAsAtomicUnit=on
  StopReason : Outport
  CANStopReason : Outport  Port=2
  wires:
  Timeout/1 -> StopFunction/2(Timeout)
  ComStop/1 -> StopFunction/1(ComStop)
  StopFunction/1(StopReason) -> StopReason/1
  ComCANStop/1 -> StopFunction/3(ComCANStop)
  StopFunction/2(CANStopReason) -> CANStopReason/1

== system Appl_HeatAdj_CtrlModel/LogicCtrl/LocalAdjustCtrl/LimitDeal/StopFunction2 ==
  ComStop : Inport
  Timeout : Inport  Port=2
  ComCANStop : Inport  Port=3  OutDataTypeStr=Enum: enHeatStopReason
  f : TriggerPort  TriggerType=function-call  VariantControl=(inherit)
      settings: CopyFcn=Stateflow.SLINSF.SimulinkMan.removeBlockPreDeleteFcn  PreDeleteFcn=Stateflow.SLINSF.SimulinkMan.unsafePredeleteFcn
  StopFunction : Stateflow chart  TreatAsAtomicUnit=on
  StopReason : Outport
  CANStopReason : Outport  Port=2
  wires:
  Timeout/1 -> StopFunction/2(Timeout)
  ComStop/1 -> StopFunction/1(ComStop)
  StopFunction/1(StopReason) -> StopReason/1
  ComCANStop/1 -> StopFunction/3(ComCANStop)
  StopFunction/2(CANStopReason) -> CANStopReason/1

== system Appl_HeatAdj_CtrlModel/LogicCtrl/LocalAdjustCtrl/LimitDeal/TimeoutFunction ==
  TimeoutPrm : Inport
  MaxTime : Inport  Port=2  OutDataTypeStr=uint32
  InLevel : Inport  Port=3
  f : TriggerPort  TriggerType=function-call  VariantControl=(inherit)
      settings: CopyFcn=Stateflow.SLINSF.SimulinkMan.removeBlockPreDeleteFcn  PreDeleteFcn=Stateflow.SLINSF.SimulinkMan.unsafePredeleteFcn
  Timeout : Stateflow chart  TreatAsAtomicUnit=on
  Level : Outport
  TimeoutFlag : Outport  Port=2
  wires:
  TimeoutPrm/1 -> Timeout/1(TimeoutPrm)
  InLevel/1 -> Timeout/2(InLevel)
  Timeout/2(Level) -> Level/1
  Timeout/1(TimeoutFlag) -> TimeoutFlag/1
  MaxTime/1 -> Timeout/3(MaxTime)

== system Appl_HeatAdj_CtrlModel/LogicCtrl/LocalAdjustCtrl/LimitDeal/TimeoutFunction1 ==
  TimeoutPrm : Inport
  MaxTime : Inport  Port=2  OutDataTypeStr=uint32
  InLevel : Inport  Port=3
  f : TriggerPort  TriggerType=function-call  VariantControl=(inherit)
      settings: CopyFcn=Stateflow.SLINSF.SimulinkMan.removeBlockPreDeleteFcn  PreDeleteFcn=Stateflow.SLINSF.SimulinkMan.unsafePredeleteFcn
  Timeout : Stateflow chart  TreatAsAtomicUnit=on
  Level : Outport
  TimeoutFlag : Outport  Port=2
  wires:
  TimeoutPrm/1 -> Timeout/1(TimeoutPrm)
  InLevel/1 -> Timeout/2(InLevel)
  Timeout/2(Level) -> Level/1
  Timeout/1(TimeoutFlag) -> TimeoutFlag/1
  MaxTime/1 -> Timeout/3(MaxTime)

== system Appl_HeatAdj_CtrlModel/LogicCtrl/LocalAdjustCtrl/LimitDeal/TimeoutFunction2 ==
  TimeoutPrm : Inport
  MaxTime : Inport  Port=2  OutDataTypeStr=uint32
  InLevel : Inport  Port=3
  SwTimeout : Inport  Port=4  OutDataTypeStr=uint32
  f : TriggerPort  TriggerType=function-call  VariantControl=(inherit)
      settings: CopyFcn=Stateflow.SLINSF.SimulinkMan.removeBlockPreDeleteFcn  PreDeleteFcn=Stateflow.SLINSF.SimulinkMan.unsafePredeleteFcn
  Timeout : Stateflow chart  TreatAsAtomicUnit=on
  Level : Outport
  TimeoutFlag : Outport  Port=2
  wires:
  TimeoutPrm/1 -> Timeout/1(TimeoutPrm)
  InLevel/1 -> Timeout/2(InLevel)
  Timeout/2(Level) -> Level/1
  Timeout/1(TimeoutFlag) -> TimeoutFlag/1
  MaxTime/1 -> Timeout/3(MaxTime)
  SwTimeout/1 -> Timeout/4(SwTimeout)

== system Appl_HeatAdj_CtrlModel/LogicCtrl/LocalAdjustCtrl/OutputDeal/HeatOutFunction ==
  SetTemp : Inport
  CurrentTemp : Inport  Port=2
  HeatLvl : Inport  Port=3
  f : TriggerPort  TriggerType=function-call  VariantControl=(inherit)
      settings: CopyFcn=Stateflow.SLINSF.SimulinkMan.removeBlockPreDeleteFcn  PreDeleteFcn=Stateflow.SLINSF.SimulinkMan.unsafePredeleteFcn
  HeatOut : Stateflow chart  TreatAsAtomicUnit=on
  HeatOutGpio : Outport
  HeatOutPwmCnt : Outport  Port=2
  wires:
  CurrentTemp/1 -> HeatOut/1(CurrentTemp)
  SetTemp/1 -> HeatOut/3(SetTemp)
  HeatLvl/1 -> HeatOut/2(HeatLvl)
  HeatOut/1(HeatOutGpio) -> HeatOutGpio/1
  HeatOut/2(HeatOutPwmCnt) -> HeatOutPwmCnt/1

== system Appl_HeatAdj_CtrlModel/LogicCtrl/LocalAdjustCtrl/OutputDeal/HeatOutFunction1 ==
  SetTemp : Inport
  CurrentTemp : Inport  Port=2
  HeatLvl : Inport  Port=3
  f : TriggerPort  TriggerType=function-call  VariantControl=(inherit)
      settings: CopyFcn=Stateflow.SLINSF.SimulinkMan.removeBlockPreDeleteFcn  PreDeleteFcn=Stateflow.SLINSF.SimulinkMan.unsafePredeleteFcn
  HeatOut : Stateflow chart  TreatAsAtomicUnit=on
  HeatOutGpio : Outport
  HeatOutPwmCnt : Outport  Port=2
  wires:
  CurrentTemp/1 -> HeatOut/1(CurrentTemp)
  SetTemp/1 -> HeatOut/3(SetTemp)
  HeatLvl/1 -> HeatOut/2(HeatLvl)
  HeatOut/1(HeatOutGpio) -> HeatOutGpio/1
  HeatOut/2(HeatOutPwmCnt) -> HeatOutPwmCnt/1

== system Appl_HeatAdj_CtrlModel/LogicCtrl/LocalAdjustCtrl/OutputDeal/HeatOutFunction2 ==
  SetTemp : Inport
  CurrentTemp : Inport  Port=2
  HeatLvl : Inport  Port=3
  MaxTime : Inport  Port=4  OutDataTypeStr=uint32
  f : TriggerPort  TriggerType=function-call  VariantControl=(inherit)
      settings: CopyFcn=Stateflow.SLINSF.SimulinkMan.removeBlockPreDeleteFcn  PreDeleteFcn=Stateflow.SLINSF.SimulinkMan.unsafePredeleteFcn
  HeatOut : Stateflow chart  TreatAsAtomicUnit=on
  HeatOutGpio : Outport
  HeatOutPwmCnt : Outport  Port=2
  SwTimeoutFlag : Outport  Port=3
  Sw20minTimer : Outport  Port=4
  wires:
  CurrentTemp/1 -> HeatOut/1(CurrentTemp)
  SetTemp/1 -> HeatOut/3(SetTemp)
  HeatLvl/1 -> HeatOut/2(HeatLvl)
  HeatOut/1(HeatOutGpio) -> HeatOutGpio/1
  HeatOut/2(HeatOutPwmCnt) -> HeatOutPwmCnt/1
  HeatOut/3(SwTimeoutFlag) -> SwTimeoutFlag/1
  HeatOut/4(Sw20minTimer) -> Sw20minTimer/1
  MaxTime/1 -> HeatOut/4(MaxTime)

== system Appl_HeatAdj_CtrlModel/LogicCtrl/LocalAdjustCtrl/OutputDeal/TempFunction ==
  AimLevel : Inport
  ProjectType : Inport  Port=2
  ThirdHeat : Inport  Port=3
  f : TriggerPort  TriggerType=function-call  VariantControl=(inherit)
      settings: CopyFcn=Stateflow.SLINSF.SimulinkMan.removeBlockPreDeleteFcn  PreDeleteFcn=Stateflow.SLINSF.SimulinkMan.unsafePredeleteFcn
  TempFunction : Stateflow chart  TreatAsAtomicUnit=on
  AimTemp : Outport
  wires:
  AimLevel/1 -> TempFunction/1(AimLevel)
  TempFunction/1(AimTemp) -> AimTemp/1
  ProjectType/1 -> TempFunction/2(ProjectType)
  ThirdHeat/1 -> TempFunction/3(ThirdHeat)

== system Appl_HeatAdj_CtrlModel/LogicCtrl/LocalAdjustCtrl/OutputDeal/TempFunction1 ==
  AimLevel : Inport
  ProjectType : Inport  Port=2
  ThirdHeat : Inport  Port=3
  f : TriggerPort  TriggerType=function-call  VariantControl=(inherit)
      settings: CopyFcn=Stateflow.SLINSF.SimulinkMan.removeBlockPreDeleteFcn  PreDeleteFcn=Stateflow.SLINSF.SimulinkMan.unsafePredeleteFcn
  TempFunction : Stateflow chart  TreatAsAtomicUnit=on
  AimTemp : Outport
  wires:
  AimLevel/1 -> TempFunction/1(AimLevel)
  TempFunction/1(AimTemp) -> AimTemp/1
  ProjectType/1 -> TempFunction/2(ProjectType)
  ThirdHeat/1 -> TempFunction/3(ThirdHeat)

== system Appl_HeatAdj_CtrlModel/LogicCtrl/LocalAdjustCtrl/OutputDeal/TempFunction2 ==
  AimLevel : Inport
  ProjectType : Inport  Port=2
  ThirdHeat : Inport  Port=3
  f : TriggerPort  TriggerType=function-call  VariantControl=(inherit)
      settings: CopyFcn=Stateflow.SLINSF.SimulinkMan.removeBlockPreDeleteFcn  PreDeleteFcn=Stateflow.SLINSF.SimulinkMan.unsafePredeleteFcn
  TempFunction : Stateflow chart  TreatAsAtomicUnit=on
  AimTemp : Outport
  wires:
  AimLevel/1 -> TempFunction/1(AimLevel)
  TempFunction/1(AimTemp) -> AimTemp/1
  ProjectType/1 -> TempFunction/2(ProjectType)
  ThirdHeat/1 -> TempFunction/3(ThirdHeat)

== system Appl_HeatAdj_CtrlModel/UpDataInputInfo/InputSignalProcess/CommonPreconditionDeal ==
  HeatAdj_PowerMode : Inport
  HeatAdj_VoltMode : Inport  Port=2
  DCDC_SwitchEnable : Inport  Port=3
  EngineRunningFlag : Inport  Port=4
  VehicleRunFlag : Inport  Port=5
  Deal : Stateflow chart  TreatAsAtomicUnit=on
  "ComPCSatisfiedFlag " : Outport
  wires:
  HeatAdj_PowerMode/1 -> Deal/1(HeatAdj_PowerMode)
  DCDC_SwitchEnable/1 -> Deal/2(DCDC_SwitchEnable)
  EngineRunningFlag/1 -> Deal/3(EngineRunningFlag)
  VehicleRunFlag/1 -> Deal/4(VehicleRunFlag)
  Deal/1(ComPCSatisfiedFlag) -> "ComPCSatisfiedFlag "/1
  HeatAdj_VoltMode/1 -> Deal/5(HeatAdj_VoltMode)

== system Appl_HeatAdj_CtrlModel/UpDataInputInfo/InputSignalProcess/DCDC_SwitchSts ==
  HeatAdj_CarType : Inport
  HeatAdj_DCDCSwitchSts : Inport  Port=2
  Constant : Constant  Value=TRUE  OutDataTypeStr=uint8
  Data Type Conversion : DataTypeConversion  OutDataTypeStr=uint8
  Switch : Switch  Criteria=u2 ~= 0
  DCDC_SwitchEnable : Outport
  wires:
  HeatAdj_CarType/1 -> Data Type Conversion/1
  HeatAdj_DCDCSwitchSts/1 -> Switch/1
  Constant/1 -> Switch/3
  Switch/1 -> DCDC_SwitchEnable/1
  Data Type Conversion/1 -> Switch/2

== system Appl_HeatAdj_CtrlModel/UpDataInputInfo/InputSignalProcess/EngineRunning ==
  HeatAdj_PlatformEngineEnableConfig : Inport
  HeatAdj_P20_PHEV_EngineCfg : Inport  Port=2
  HeatAdj_ECMD_EngineStatus : Inport  Port=3
  HeatAdj_CarType : Inport  Port=4
  EngineStatus : Stateflow chart  TreatAsAtomicUnit=on
  "EngineRunningFlag " : Outport
  wires:
  EngineStatus/1(EngineRunningFlag) -> "EngineRunningFlag "/1
  HeatAdj_ECMD_EngineStatus/1 -> EngineStatus/3(HeatAdj_ECMD_EngineStatus)
  HeatAdj_PlatformEngineEnableConfig/1 -> EngineStatus/1(HeatAdj_PlatformEngineEnableConfig)
  HeatAdj_P20_PHEV_EngineCfg/1 -> EngineStatus/2(HeatAdj_P20_PHEV_EngineCfg)
  HeatAdj_CarType/1 -> EngineStatus/4(HeatAdj_CarType)

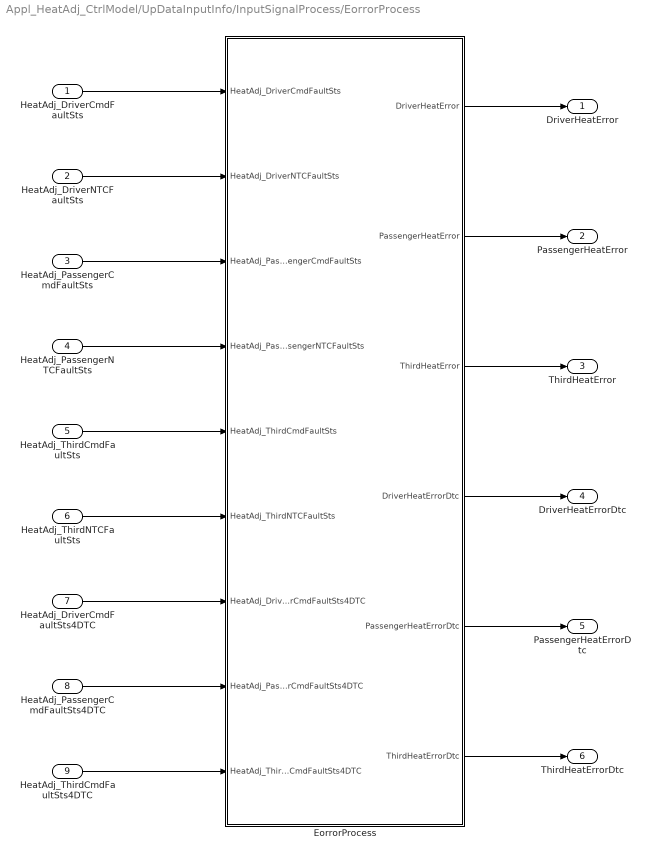
== system Appl_HeatAdj_CtrlModel/UpDataInputInfo/InputSignalProcess/EorrorProcess ==
  HeatAdj_DriverCmdFaultSts : Inport
  HeatAdj_DriverNTCFaultSts : Inport  Port=2
  HeatAdj_PassengerCmdFaultSts : Inport  Port=3
  HeatAdj_PassengerNTCFaultSts : Inport  Port=4
  HeatAdj_ThirdCmdFaultSts : Inport  Port=5
  HeatAdj_ThirdNTCFaultSts : Inport  Port=6
  HeatAdj_DriverCmdFaultSts4DTC : Inport  Port=7
  HeatAdj_PassengerCmdFaultSts4DTC : Inport  Port=8
  HeatAdj_ThirdCmdFaultSts4DTC : Inport  Port=9
  EorrorProcess : Stateflow chart  TreatAsAtomicUnit=on
  "DriverHeatError " : Outport
  "PassengerHeatError " : Outport  Port=2
  "ThirdHeatError " : Outport  Port=3
  DriverHeatErrorDtc : Outport  Port=4
  PassengerHeatErrorDtc : Outport  Port=5
  ThirdHeatErrorDtc : Outport  Port=6
  wires:
  EorrorProcess/3(ThirdHeatError) -> "ThirdHeatError "/1
  EorrorProcess/2(PassengerHeatError) -> "PassengerHeatError "/1
  EorrorProcess/1(DriverHeatError) -> "DriverHeatError "/1
  HeatAdj_ThirdNTCFaultSts/1 -> EorrorProcess/6(HeatAdj_ThirdNTCFaultSts)
  HeatAdj_ThirdCmdFaultSts/1 -> EorrorProcess/5(HeatAdj_ThirdCmdFaultSts)
  HeatAdj_PassengerNTCFaultSts/1 -> EorrorProcess/4(HeatAdj_PassengerNTCFaultSts)
  HeatAdj_PassengerCmdFaultSts/1 -> EorrorProcess/3(HeatAdj_PassengerCmdFaultSts)
  HeatAdj_DriverCmdFaultSts/1 -> EorrorProcess/1(HeatAdj_DriverCmdFaultSts)
  HeatAdj_DriverNTCFaultSts/1 -> EorrorProcess/2(HeatAdj_DriverNTCFaultSts)
  HeatAdj_DriverCmdFaultSts4DTC/1 -> EorrorProcess/7(HeatAdj_DriverCmdFaultSts4DTC)
  HeatAdj_PassengerCmdFaultSts4DTC/1 -> EorrorProcess/8(HeatAdj_PassengerCmdFaultSts4DTC)
  HeatAdj_ThirdCmdFaultSts4DTC/1 -> EorrorProcess/9(HeatAdj_ThirdCmdFaultSts4DTC)
  EorrorProcess/4(DriverHeatErrorDtc) -> DriverHeatErrorDtc/1
  EorrorProcess/5(PassengerHeatErrorDtc) -> PassengerHeatErrorDtc/1
  EorrorProcess/6(ThirdHeatErrorDtc) -> ThirdHeatErrorDtc/1
